simulink model "pendu_vesc_v2"  (R2018b)
settings: Solver=FixedStepAuto  StartTime=0.0  StopTime=inf  RelTol=1e-3  EnableMultiTasking=on
libraries: peGeneralControl x3, cm_custom x2, simulink x1
settings Model: SimulationMode=external  Creator=Ng Wee Shen  LastModifiedBy=Raymond
settings SolverCC: PositivePriorityOrder=on  AutoInsertRateTranBlk=on
settings OptimizationCC: EnhancedBackFolding=on  PassReuseOutputArgsAs=Individual arguments  MaxStackSize=64  OptimizeBlockOrder=speed  DifferentSizesBufferReuse=on
settings DebuggingCC: TimeAdjustmentMsg=warning  SingleTaskRateTransMsg=warning  ParameterTunabilityLossMsg=error  SFcnCompatibilityMsg=warning
settings HardwareCC: ProdBitPerPointer=32  ProdBitPerSizeT=32  ProdBitPerPtrDiffT=32  ProdLargestAtomicInteger=Long  ProdLargestAtomicFloat=Double  ProdWordSize=32  ProdHWDeviceType=ARM Compatible->ARM Cortex
settings SFSimCC: MATLABDynamicMemAlloc=off
settings RTWCC: SystemTargetFile=ert.tlc  HardwareBoard=Raspberry Pi  TLCOptions="-aInlineSetEventsForThisBaseRateFcn=TLC_FALSE -aSuppressMultiTaskScheduler=TLC_FALSE  -aRateBasedStepFcn=0"  TemplateMakefile=ert_default_tmf  Toolchain=GNU GCC Raspberry Pi  BuildConfiguration=Specify  IncludeHyperlinkInReport=on  TargetLang=C++
settings CodeAppCC: ForceParamTrailComments=on  IgnoreCustomStorageClasses=off  OperatorAnnotations=on  SimulinkDataObjDesc=on  SFDataObjDesc=on  InsertBlockDesc=on
settings ERTTargetCC: TargetLangStandard=C++03 (ISO)  SupportContinuousTime=on  SupportVariableSizeSignals=on  ExtMode=on  ExtModeMexArgs='192.168.0.173' 1 17725

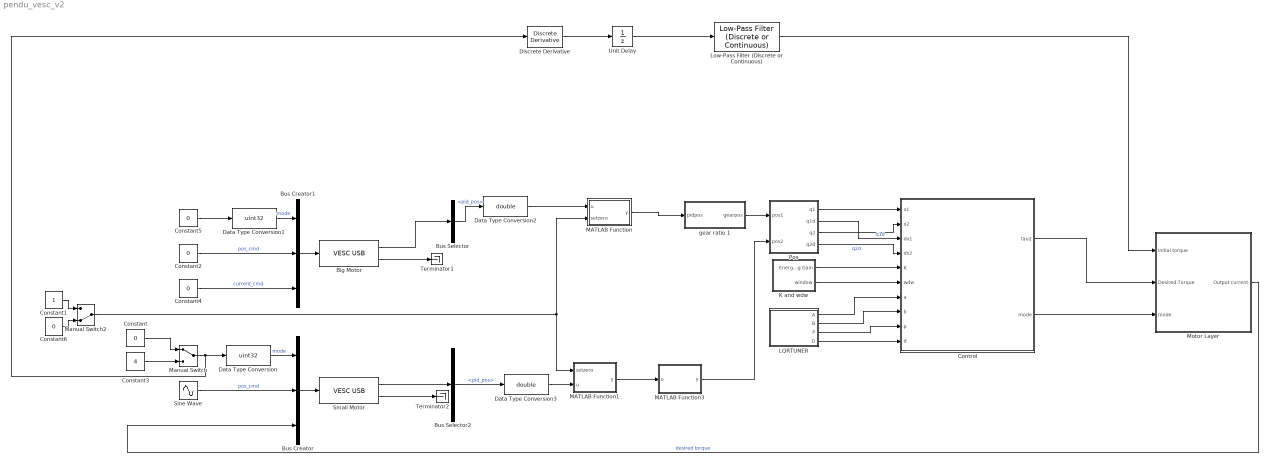
== system pendu_vesc_v2 ==
  Big Motor : cm_custom/VESC USB  PAR_VESC_DEV='/dev/VESC_BIG'  POS_KP=0.03  POS_KI=0  POS_KD=0.0004  POS_KD_FIL=0.2  POS_DIV=1  CURR_MAX=5  CURR_MIN=-5  CURR_IN_MAX=99  CURR_IN_MIN=-60  CURR_ABS_MAX=130  PAR_SMPLT=0.0025
      settings: SourceProductName=cm custom
  Bus Creator : BusCreator  Inputs=3
  Bus Creator1 : BusCreator  Inputs=3
  Bus Selector : BusSelector  OutputSignals=pid_pos
  Bus Selector2 : BusSelector  OutputSignals=pid_pos
  Constant{,2,4..6} (5 alike) : Constant  Value=0
  Constant1 : Constant
  Constant3 : Constant  Value=4
  Control : MATLAB Function  TreatAsAtomicUnit=on
  Data Type Conversion : DataTypeConversion  OutDataTypeStr=uint32
  Data Type Conversion1 : DataTypeConversion  OutDataTypeStr=uint32
  Data Type Conversion2 : DataTypeConversion  OutDataTypeStr=double
  Data Type Conversion3 : DataTypeConversion  OutDataTypeStr=double
  Discrete Derivative : simulink/Discrete/Discrete Derivative  gainval=1.0  ICPrevScaledInput=0.0  OutMin=[]  OutMax=[]  OutDataType=fixdt(1, 16)  OutScaling=2^-10  DoSatur=off
  K and wdw : Subsystem
  LQRTUNER : Subsystem
  Low-Pass Filter (Discrete or Continuous) : peGeneralControl/Low-Pass Filter (Discrete or Continuous)  K=-1  T=0.025  B=0.05  A=-0.05  Ts=-1
  MATLAB Function : MATLAB Function  TreatAsAtomicUnit=on
  MATLAB Function1 : MATLAB Function  TreatAsAtomicUnit=on
  MATLAB Function3 : MATLAB Function  TreatAsAtomicUnit=on
  Manual Switch : ManualSwitch
  Manual Switch2 : ManualSwitch  CurrentSetting=0
  Motor Layer : Subsystem
  Pos : Subsystem
  Sine Wave : Sin  Amplitude=150  Bias=10  SampleTime=0
  Small Motor : cm_custom/VESC USB  PAR_VESC_DEV='/dev/VESC_SMALL'  POS_KP=0.03  POS_KI=0  POS_KD=0.0004  POS_KD_FIL=0.2  POS_DIV=1  CURR_MAX=15  CURR_MIN=-15  CURR_IN_MAX=99  CURR_IN_MIN=-60  CURR_ABS_MAX=130  PAR_SMPLT=0.0025
      settings: SourceProductName=cm custom
  Terminator1 : Terminator
  Terminator2 : Terminator
  Unit Delay : UnitDelay  SampleTime=-1
  gear ratio 1 : Subsystem
  wires:
  Big Motor/1 -> Bus Selector/1
  Big Motor/2 -> Terminator1/1
  Data Type Conversion/1 -> Bus Creator/1  "mode"
  Bus Selector/1 -> Data Type Conversion2/1  "<pid_pos>"
  Constant3/1 -> Manual Switch/2
  Constant/1 -> Manual Switch/1
  Sine Wave/1 -> Bus Creator/2  "pos_cmd"
  Constant4/1 -> Bus Creator1/3  "current_cmd"
  Data Type Conversion1/1 -> Bus Creator1/1  "mode"
  Constant2/1 -> Bus Creator1/2  "pos_cmd"
  Constant5/1 -> Data Type Conversion1/1
  Bus Selector2/1 -> Data Type Conversion3/1  "<pid_pos>"
  Small Motor/1 -> Bus Selector2/1
  Small Motor/2 -> Terminator2/1
  Pos/2(q1d) -> Control/3(dx1)  "q1d"
  K and wdw/1(EnergyShaping Gain) -> Control/5(K)
  K and wdw/2(window) -> Control/6(wdw)
  LQRTUNER/3(P) -> Control/9(p)
  LQRTUNER/4(D) -> Control/10(d)
  LQRTUNER/2(B) -> Control/8(b)
  LQRTUNER/1(A) -> Control/7(a)
  Data Type Conversion3/1 -> MATLAB Function1/2(u)
  Constant1/1 -> Manual Switch2/1
  Constant6/1 -> Manual Switch2/2
  Manual Switch2/1 -> MATLAB Function/2(setzero), MATLAB Function1/1(setzero)
  Manual Switch/1 -> Data Type Conversion/1, Discrete Derivative/1
  Discrete Derivative/1 -> Unit Delay/1
  Unit Delay/1 -> Low-Pass Filter (Discrete or Continuous)/1
  Low-Pass Filter (Discrete or Continuous)/1 -> Motor Layer/1(initial torque)
  Pos/1(q1) -> Control/1(x1)
  Pos/3(q2) -> Control/2(x2)
  Bus Creator/1 -> Small Motor/1
  Bus Creator1/1 -> Big Motor/1
  Pos/4(q2d) -> Control/4(dx2)  "q2d"
  Control/2(mode) -> Motor Layer/3(" mode ")
  Control/1(tau2) -> Motor Layer/2(Desired Torque)
  Data Type Conversion2/1 -> MATLAB Function/1(u)
  MATLAB Function/1(y) -> gear ratio 1/1(pidpos)
  gear ratio 1/1(gearpos) -> Pos/1(pos1)
  MATLAB Function1/1(y) -> MATLAB Function3/1(u)
  MATLAB Function3/1(y) -> Pos/2(pos2)
  Motor Layer/1(Output current) -> Bus Creator/3  "desired torque"

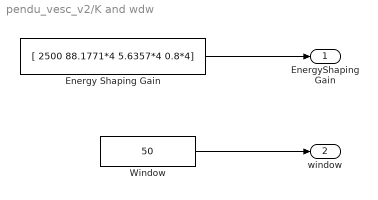
== system pendu_vesc_v2/K and wdw ==
  Energy Shaping Gain : Constant  Value=[ 2500 88.1771*4 5.6357*4 0.8*4]
  Window : Constant  Value=50
  EnergyShaping Gain : Outport
  window : Outport  Port=2
  wires:
  Energy Shaping Gain/1 -> EnergyShaping Gain/1
  Window/1 -> window/1

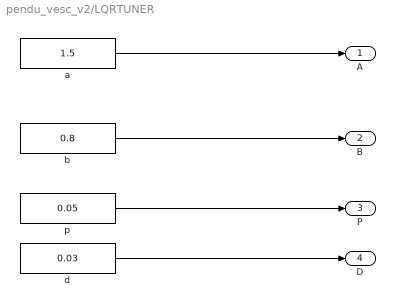
== system pendu_vesc_v2/LQRTUNER ==
  a : Constant  Value=1.5
  b : Constant  Value=0.8
  d : Constant  Value=0.03
  p : Constant  Value=0.05
  A : Outport
  B : Outport  Port=2
  P : Outport  Port=3
  D : Outport  Port=4
  wires:
  p/1 -> P/1
  b/1 -> B/1
  d/1 -> D/1
  a/1 -> A/1

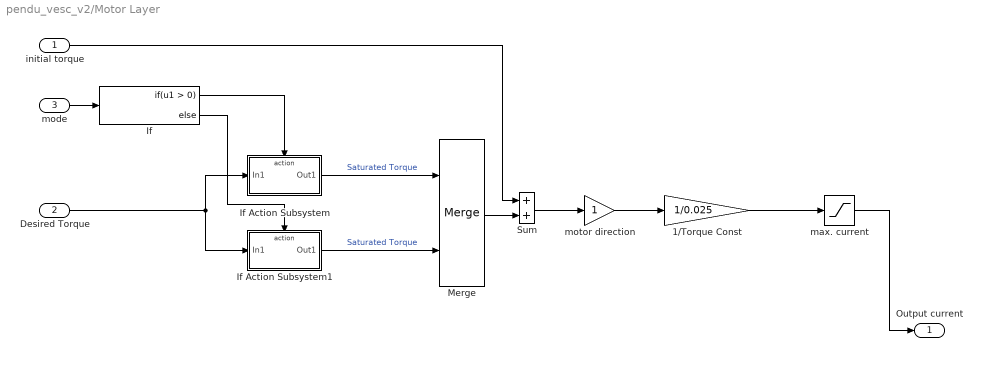
== system pendu_vesc_v2/Motor Layer ==
  initial torque : Inport
  Desired Torque : Inport  Port=2
  " mode " : Inport  Port=3
  1/Torque Const : Gain  Gain=1/0.025  OutDataTypeStr=Inherit: Same as input
  If : If
  If Action Subsystem : Subsystem  TreatAsAtomicUnit=on
  If Action Subsystem1 : Subsystem  TreatAsAtomicUnit=on
  Merge : Merge
  Sum : Sum
  max. current : Saturate  UpperLimit=5  LowerLimit=-5  LinearizeAsGain=off
  motor direction : Gain  OutDataTypeStr=Inherit: Same as input
  Output current : Outport
  wires:
  motor direction/1 -> 1/Torque Const/1
  max. current/1 -> Output current/1
  " mode "/1 -> If/1
  Desired Torque/1 -> If Action Subsystem/1(In1), If Action Subsystem1/1(In1)
  If Action Subsystem/1(Out1) -> Merge/1  "Saturated Torque"
  If Action Subsystem1/1(Out1) -> Merge/2  "Saturated Torque"
  If/1 -> If Action Subsystem/Action
  If/2 -> If Action Subsystem1/Action
  Merge/1 -> Sum/2
  Sum/1 -> motor direction/1
  initial torque/1 -> Sum/1
  1/Torque Const/1 -> max. current/1

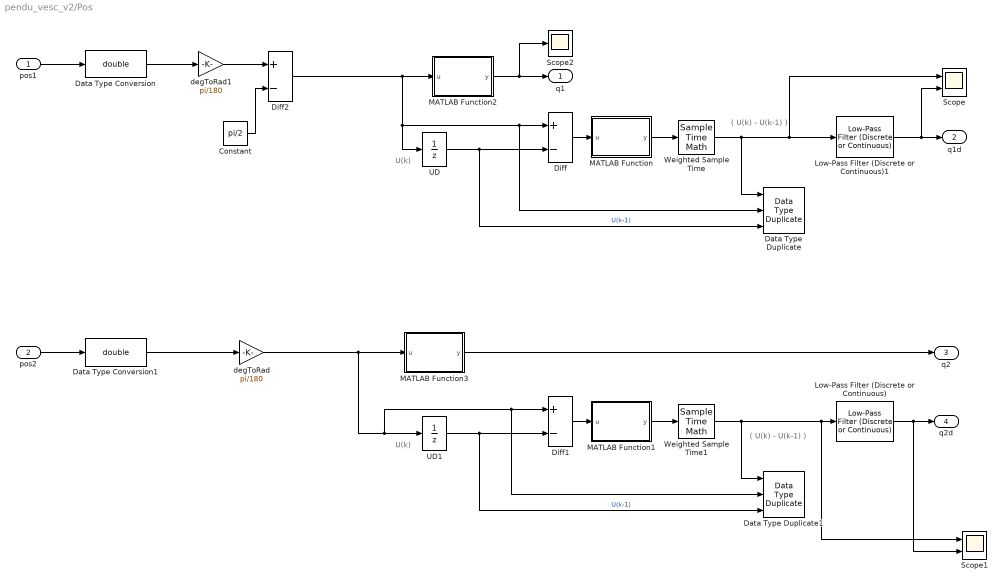
== system pendu_vesc_v2/Pos ==
  note: ( U(k) - U(k-1) )
  note: U(k)
  note: U(k)
  note: ( U(k) - U(k-1) )
  pos1 : Inport
  pos2 : Inport  Port=2
  Constant : Constant  Value=pi/2
  Data Type Duplicate : DataTypeDuplicate  DisableCoverage=on  NumInputPorts=3
  Data Type Duplicate1 : DataTypeDuplicate  DisableCoverage=on  NumInputPorts=3
  Data Type Conversion : DataTypeConversion  OutDataTypeStr=double
  Data Type Conversion1 : DataTypeConversion  OutDataTypeStr=double
  Diff : Sum  Description=Add in CPU  Inputs=+-
  Diff1 : Sum  Description=Add in CPU  Inputs=+-
  Diff2 : Sum  Description=Add in CPU  Inputs=+-
  Low-Pass Filter (Discrete or Continuous) : peGeneralControl/Low-Pass Filter (Discrete or Continuous)  K=1  T=0.02  B=inf  A=-inf  Ts=-1
  Low-Pass Filter (Discrete or Continuous)1 : peGeneralControl/Low-Pass Filter (Discrete or Continuous)  K=1  T=0.02  B=inf  A=-inf  Ts=-1
  MATLAB Function : MATLAB Function  TreatAsAtomicUnit=on
  MATLAB Function1 : MATLAB Function  TreatAsAtomicUnit=on
  MATLAB Function2 : MATLAB Function  TreatAsAtomicUnit=on
  MATLAB Function3 : MATLAB Function  TreatAsAtomicUnit=on
  Scope : Scope  NumInputPorts=2
  Scope1 : Scope  NumInputPorts=2
  Scope2 : Scope
  UD : UnitDelay  Description=Store in Global RAM  DisableCoverage=on  SampleTime=-1
  UD1 : UnitDelay  Description=Store in Global RAM  DisableCoverage=on  SampleTime=-1
  Weighted Sample Time : SampleTimeMath  TsampMathOp=/
  Weighted Sample Time1 : SampleTimeMath  TsampMathOp=/
  degToRad : Gain  Gain=pi/180
  degToRad1 : Gain  Gain=pi/180
  q1 : Outport
  q1d : Outport  Port=2
  q2 : Outport  Port=3
  q2d : Outport  Port=4
  wires:
  pos2/1 -> Data Type Conversion1/1
  pos1/1 -> Data Type Conversion/1
  Data Type Conversion/1 -> degToRad1/1
  Diff/1 -> MATLAB Function/1(u)
  UD/1 -> Diff/2, Data Type Duplicate/3  "U(k-1)"
  MATLAB Function/1(y) -> Weighted Sample Time/1
  Weighted Sample Time/1 -> Data Type Duplicate/1, Scope/1, Low-Pass Filter (Discrete or Continuous)1/1
  UD1/1 -> Diff1/2, Data Type Duplicate1/3  "U(k-1)"
  Diff1/1 -> MATLAB Function1/1(u)
  MATLAB Function1/1(y) -> Weighted Sample Time1/1
  Low-Pass Filter (Discrete or Continuous)1/1 -> Scope/2, q1d/1
  degToRad1/1 -> Diff2/1
  Constant/1 -> Diff2/2
  Diff2/1 -> MATLAB Function2/1(u), Data Type Duplicate/2, Diff/1, UD/1
  MATLAB Function2/1(y) -> Scope2/1, q1/1
  MATLAB Function3/1(y) -> q2/1
  degToRad/1 -> MATLAB Function3/1(u), UD1/1, Diff1/1, Data Type Duplicate1/2
  Data Type Conversion1/1 -> degToRad/1
  Low-Pass Filter (Discrete or Continuous)/1 -> Scope1/2, q2d/1
  Weighted Sample Time1/1 -> Data Type Duplicate1/1, Scope1/1, Low-Pass Filter (Discrete or Continuous)/1

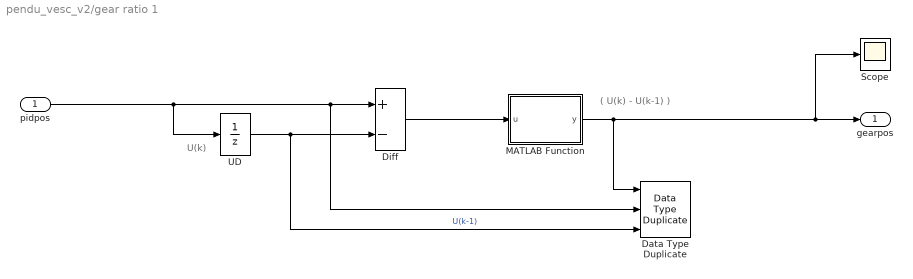
== system pendu_vesc_v2/gear ratio 1 ==
  note: ( U(k) - U(k-1) )
  note: U(k)
  pidpos : Inport
  Data Type Duplicate : DataTypeDuplicate  DisableCoverage=on  NumInputPorts=3
  Diff : Sum  Description=Add in CPU  Inputs=+-
  MATLAB Function : MATLAB Function  TreatAsAtomicUnit=on
  Scope : Scope
  UD : UnitDelay  Description=Store in Global RAM  DisableCoverage=on  SampleTime=-1
  gearpos : Outport
  wires:
  UD/1 -> Diff/2, Data Type Duplicate/3  "U(k-1)"
  pidpos/1 -> UD/1, Diff/1, Data Type Duplicate/2
  MATLAB Function/1(y) -> Data Type Duplicate/1, Scope/1, gearpos/1
  Diff/1 -> MATLAB Function/1(u)

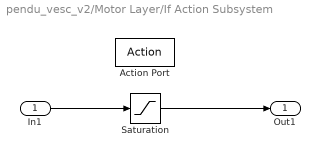
== system pendu_vesc_v2/Motor Layer/If Action Subsystem ==
  In1 : Inport
  Action Port : ActionPort  ActionType=then
  Saturation : Saturate  UpperLimit=0.35  LowerLimit=-0.35
  Out1 : Outport
  wires:
  In1/1 -> Saturation/1
  Saturation/1 -> Out1/1

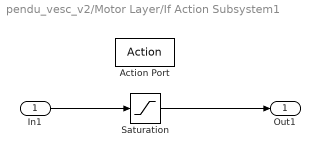
== system pendu_vesc_v2/Motor Layer/If Action Subsystem1 ==
  In1 : Inport
  Action Port : ActionPort  ActionType=else
  Saturation : Saturate  UpperLimit=0.35  LowerLimit=-0.35
  Out1 : Outport
  wires:
  In1/1 -> Saturation/1
  Saturation/1 -> Out1/1

== matlab function pendu_vesc_v2/MATLAB Function ==
  data: u input; setzero input; y output
function y = fcn(u,setzero)

persistent initpos
if isempty(initpos)
    initpos = 0;
end

if setzero
    initpos = u + 0;
end
x = u - initpos;
y = (-x + 360)*(x>0) + (-x)*(x<0);

== matlab function pendu_vesc_v2/Control ==
  data: x1 input; x2 input; dx1 input; dx2 input; K input; wdw input; a input; b input; p input; d input; tau2 output; mode output
function [tau2,mode] = EnergyShaping_w_LQR(x1,x2,dx1,dx2,K,wdw,a,b,p,d)
% Match the setup in simulation

Kv = K(1);
Kp = K(2);
Kd = K(3);
Ke = K(4);
x = [x1;x2;dx1;dx2]; 

persistent model;
if isempty(model)
    model = Model();
end
%%%%
q  = x(1:2,:);
q(1) = q(1)- 2*pi*floor((q(1)+pi)./(2*pi));
qd = x(3:4,:);
g  = model.g;
%
l1 = model.l1; lc1 = model.lc1; 
l2 = model.l2; lc2 = model.lc2;
m1 = model.m1; m2 = model.m2;
I1 = model.I1; I2 = model.I2;
b1 = model.b1; b2 = model.b2;
%
s = sin(q(1:2));
s12 = sin(q(1)+q(2));

[M, C, G, ~,~,~] = ManipulatorEquation(model, x);
[tau,mode] = acrobotControlLaw_LQR(x,wdw,a,b,p,d,model);

% compute energy
ke = 0.5*qd'*M*qd;
pe = (m1*lc1+m2*l1)*g*(s(1)-1)+m2*g*lc2*(s12-1);
E = ke + pe;
dem = 1;
delta = 1;
if isempty(tau) % if LQR control law is not applicable, 
                %    then using Energy Shaping approach
    mode = 0;

    d11 = M(1,1);
    d12 = M(1,2);
    d21 = M(2,1);
    d22 = M(2,2);
    delta = d11*d22-d21*d12;
    
    H = C*qd;
    
    h1 = H(1);
    h2 = H(2);
    p1 = G(1);
    p2 = G(2);
    
    dem = Ke*E*delta+Kd*d11;
    tau2 = -delta*(Kv*qd(2)+Kp*q(2))/dem - (Kd*d21*(h1+p1)+Kd*d11*(h2+p2))/dem;
    tau = [0;tau2]/3;
    if abs(tau2) >= 0.3
        tau2 = 0.3 * sign(tau2);
    end
    tau = [0;0];
end
tau1 = tau(1);
tau2 = tau(2);
tau = [0;tau2];
end

== matlab function pendu_vesc_v2/MATLAB Function1 ==
  data: setzero input; u input; y output
function y = fcn(setzero,u)

persistent initpos
if isempty(initpos)
    initpos = 0;
end

if setzero
    initpos = u + 0;
end


y = u - initpos;
y = y - 360*floor(y/360);

== matlab function pendu_vesc_v2/Pos/MATLAB Function ==
  data: u input; y output
function y = fcn(u)

u_rev = (u >= 0)*(2*pi - u) + (u < 0)*(2*pi + u);

if abs(u_rev) > abs(u)
   y = u;
else
   y = (u < 0)*u_rev - (u >= 0)*u_rev;
end

== matlab function pendu_vesc_v2/Pos/MATLAB Function1 ==
  data: u input; y output
function y = fcn(u)

u_rev = (u >= 0)*(2*pi - u) + (u < 0)*(2*pi + u);

if abs(u_rev) > abs(u)
   y = u;
else
   y = (u < 0)*u_rev - (u >= 0)*u_rev;
end

== matlab function pendu_vesc_v2/Pos/MATLAB Function2 ==
  data: u input; y output
function y = fcn(u)
    y = u - 2*pi*floor((u + pi)./(2*pi));
end

== matlab function pendu_vesc_v2/Pos/MATLAB Function3 ==
  data: u input; y output
function y = fcn(u)
    y = u - 2*pi*floor((u + pi)/(2*pi));
end

== matlab function pendu_vesc_v2/gear ratio 1/MATLAB Function ==
  data: u input; y output
function y = fcn(u)

% first joint
gear_ratio = (90/26);
persistent pos1
if isempty(pos1)
    pos1 = 0;
end

u_rev = (u >= 0)*(360 - u) + (u < 0)*(360 + u);
if abs(u_rev) < abs(u)
   u = (u < 0)*u_rev - (u >= 0)*u_rev;
end

u = u/gear_ratio;
pos1 = pos1 + u;
pos1 = mod((pos1),360);
y = pos1;

end

== matlab function pendu_vesc_v2/MATLAB Function3 ==
  data: u input; y output
function y = fcn(u)
% u --> q1
y = (-u + 360)*(u>0) + (-u)*(u<0);
end
